simulink model "CONTROL_SYSTEM_V2"  (R2024a)
settings: Solver=ode1  StartTime=0.0  StopTime=inf  FixedStep=0.01  RelTol=1e-5
values from neighbouring files (symbols this model uses):
  B_aet = 0.1503    [System_Setting.m]
  Beta1 = 3*Omega_o    (= 750)    [Control_Setting.m]
  Beta2 = 3*(Omega_o^2)    (= 187500)    [Control_Setting.m]
  Beta3 = (Omega_o^3)    (= 15625000)    [Control_Setting.m]
  F_so = 0.089    [System_Setting.m]
  J_aet = 0.0035    [System_Setting.m]
  K_sp = 0.0914    [System_Setting.m]
  omga_c = 100    [Control_Setting.m]
  roa = 0.24    [System_Setting.m]
  theta_o = 12    [System_Setting.m]
  Toa_ho = 0.3193    [System_Setting.m]
undefined symbols (not defined in the file or in its folder): Desire_Max, Desire_Min, Direction_Pin, EN_Pin, Kd, Ki, Kn, Kp, sigbuilder_block
libraries: arduinolib x29, simulink_extras x12, slpidlib x3, spsOnDelayLib x2, simulink x2, slctrl_autotuning x2
(part 1 of 3)
settings Model: NumberOfSteps=2  ExtModeTrigDuration=2  Creator=Banana444  LastModifiedBy=Banana444
settings SolverCC: ZeroCrossAlgorithm=Adaptive  AutoInsertRateTranBlk=on
settings OptimizationCC: EnhancedBackFolding=on  PassReuseOutputArgsAs=Individual arguments  ZeroExternalMemoryAtStartup=off  ZeroInternalMemoryAtStartup=off  MaxStackSize=64  OptimizeBlockOrder=speed  DifferentSizesBufferReuse=on  OptimizationCustomize=off  EfficientTunableParamExpr=on
settings DebuggingCC: IgnoredZcDiagnostic=none  ParameterTunabilityLossMsg=error
settings HardwareCC: ProdBitPerPointer=32  ProdBitPerSizeT=32  ProdBitPerPtrDiffT=32  ProdLargestAtomicInteger=Long  ProdLargestAtomicFloat=Double  ProdWordSize=32  ProdHWDeviceType=ARM Compatible->ARM Cortex
settings SFSimCC: MATLABDynamicMemAlloc=off
settings RTWCC: Description=Embedded Coder  SystemTargetFile=ert.tlc  HardwareBoard=ESP32-WROOM(Arduino Compatible)  TLCOptions="-aInlineSetEventsForThisBaseRateFcn=TLC_FALSE -aSuppressMultiTaskScheduler=TLC_FALSE  -aRateBasedStepFcn=0"  TemplateMakefile=ert_default_tmf  Toolchain=ESP32
settings CodeAppCC: ForceParamTrailComments=on  IgnoreCustomStorageClasses=off  OperatorAnnotations=on  SimulinkDataObjDesc=on  SFDataObjDesc=on  InsertBlockDesc=on
settings ERTTargetCC: SupportContinuousTime=on  SupportVariableSizeSignals=on  ExtModeTransport=3  ExtModeStaticAlloc=on  ExtModeAutomaticAllocSize=off  ExtModeStaticAllocSize=65536  ExtModeMexFile=ext_xcp  ExtModeIntrfLevel=Level2 - Open

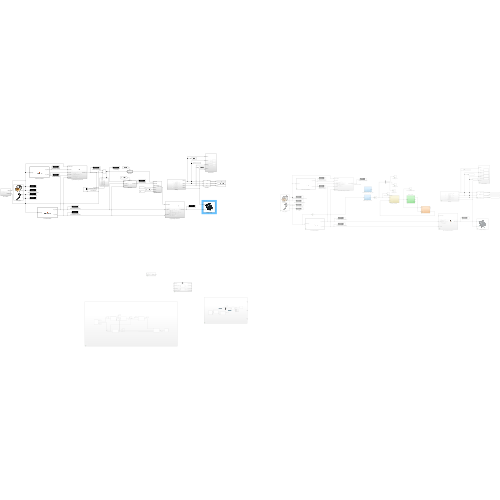
[thumbnail: Simulink's stored preview of the top-level diagram]
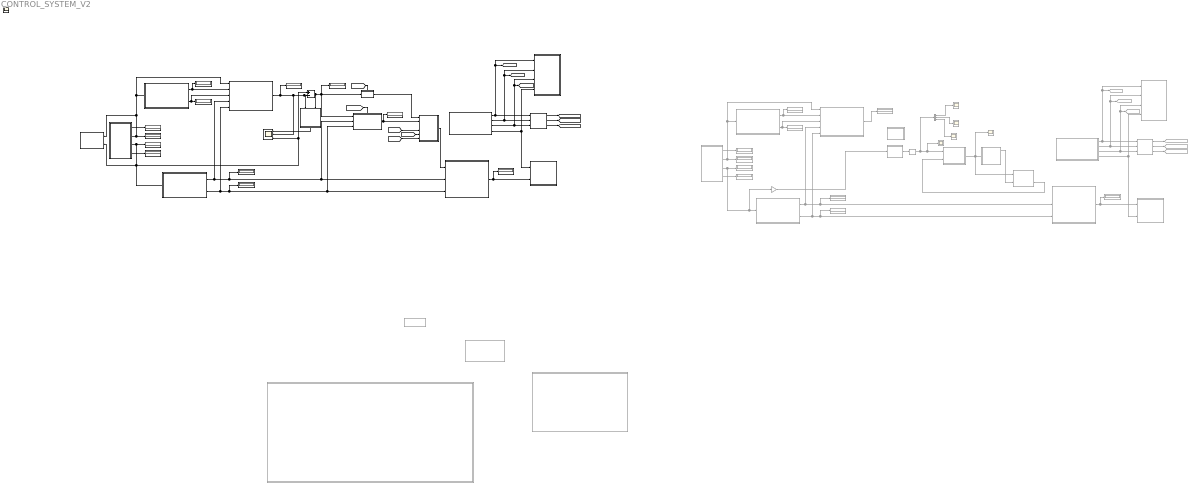
== system CONTROL_SYSTEM_V2 ==
  AETV_system : Subsystem  Commented=on
  Analog Signal : Subsystem
      mask Display: image('Capture.JPG');
  Analog Signal1 : Subsystem  Commented=on
      mask Display: image('Capture.JPG');
  Button Control : Subsystem
  Button Control1 : Subsystem  Commented=on
  Contro_input (Voltages) : Scope  Commented=on
  Contro_input (Voltages)1 : Scope  Commented=on
  Degrees to Radians1 : simulink_extras/Transformations/Degrees to Radians  Commented=on
  Demux : Demux  Commented=on  Outputs=3
  Desired signals_Sinewave : Subsystem  Commented=on
  Desired_Reference_step_input : Subsystem  Commented=on
  Display1 : Display  Commented=on
      settings: Decimation=2
  Display3 : Display
      settings: Decimation=2
  Error Indication : Subsystem
      settings: PortSchema="{\"entries\":[{\"content\":{\"sides\":[{\"content\":{},\"type\":\"ConnectorPlacement.EquallySpacedRectSide\",\"uuid\":\"6bb27259-0fc4-412b-bd28-187413250838\"},{\"content\":{\"connectorIds\":[\"In1\",\"In2\"],\"side\":\"RIGHT\"},\"type\":\"ConnectorPlacement.EquallySpacedRectSide\",\"uuid\":\"b38a583a-7cdb-4b72-8a0e-445370b0f03f\"},{\"content\":{\"side\":\"TOP\"},\"type\":\"ConnectorPlacement.EquallySpacedRectSide\",\"uuid\":\"477ad40e-8e68-4653-afaf-50b4ab734c9d\"}]},\"type\":\"ConnectorPlacement.EquallySpacedConnector\",\"uuid\":\"474c0f68-6b48-44ee-b6ec-af4e49acdc40\"}],\"packageUris\":[\"http://schema.mathworks.com/mf0/Connector/R2020b\"],\"version\":\"1.0\"}"
  Error Reading : Display
      settings: Decimation=2
  FP_Input Range Conversion : Subsystem
  FP_Input Range Conversion1 : Subsystem  Commented=on
  Foot Pedal Calibration : MATLAB Function  TreatAsAtomicUnit=on
  Foot Pedal Calibration1 : MATLAB Function  Commented=on  TreatAsAtomicUnit=on
  Foot Pedal Maximum Reading : Display
      settings: Decimation=2
  Foot Pedal Maximum Reading1 : Display  Commented=on
      settings: Decimation=2
  Foot Pedal Minimum Reading : Display
      settings: Decimation=2
  Foot Pedal Minimum Reading1 : Display  Commented=on
      settings: Decimation=2
  Foot Pedal Reading : Display
      settings: Decimation=2
  Foot Pedal Reading1 : Display  Commented=on
      settings: Decimation=2
  Foot Pedal Signal VS Throttle Body Position : Scope  NumInputPorts=3
  Goto10 : Goto  Commented=on  GotoTag=Button_2
  Goto11 : Goto  Commented=on  GotoTag=Button_3
  Goto6 : Goto  Commented=on  GotoTag=No_Control
  Goto7 : Goto  Commented=on  GotoTag=PID_Control
  Goto8 : Goto  Commented=on  GotoTag=Advance_Control
  Goto9 : Goto  Commented=on  GotoTag=Button_1
  H-Bridge Setting : Subsystem
      mask Display: image('H-Bridge-removebg-preview.png');
  H-Bridge Setting1 : Subsystem  Commented=on
      mask Display: image('H-Bridge-removebg-preview.png');
  If Condition : If  NumInputs=3  IfExpression=u1 == 1  ElseIfExpressions=u2 == 1, u3 == 1  ShowElse=off
  If Condition1 : If  Commented=on  NumInputs=3  IfExpression=u1 == 1  ElseIfExpressions=u2 == 1, u3 == 1  ShowElse=off
  Latching : Subsystem
  Latching1 : Subsystem  Commented=on
  Multiply : Gain  Commented=on  Gain=10
  NaN : Display
      settings: Decimation=2
  NaN1 : Display  Commented=on
      settings: Decimation=2
  No Control : Subsystem  TreatAsAtomicUnit=on
  Operation Selector : Subsystem
  PID Control : Subsystem
  PID Output Reading : Display
      settings: Decimation=2
  SFBC_Controller : Subsystem  Commented=on
  Subsystem : Subsystem
      settings: PortSchema="{\"entries\":[{\"content\":{\"sides\":[{\"content\":{},\"type\":\"ConnectorPlacement.EquallySpacedRectSide\",\"uuid\":\"06ab9b8c-dc11-4e78-9aea-2a49b899d383\"},{\"content\":{\"side\":\"RIGHT\"},\"type\":\"ConnectorPlacement.EquallySpacedRectSide\",\"uuid\":\"ea81575a-6f3e-44ea-98d6-a15110b05ea2\"},{\"content\":{\"connectorIds\":[\"In1\",\"In2\"],\"side\":\"TOP\"},\"type\":\"ConnectorPlacement.EquallySpacedRectSide\",\"uuid\":\"b4582e74-93d2-4cba-bd7b-a3215d2fef1c\"},{\"content\":{\"connectorIds\":[\"Out1\"],\"side\":\"BOTTOM\"},\"type\":\"ConnectorPlacement.EquallySpacedRectSide\",\"uuid\":\"d3012ec7-4a68-4cee-bd0d-e63c4f089545\"}]},\"type\":\"ConnectorPlacement.EquallySpacedConnector\",\"uuid\":\"85ff3d74-6a46-44e9-8a38-f9999c5d3ee8\"}],\"packageUris\":[\"http://schema.mathworks.com/mf0/Connector/R2020b\"],\"version\":\"1.0\"}"
  Subsystem1 : Subsystem  Commented=on
  Subsystem2 : Subsystem  Commented=on
  Subsystem4 : Subsystem  Commented=on
  Subsystem5 : Subsystem  Commented=on
  Subsystem6 : Subsystem  Commented=on
  Sum2 : Sum  Inputs=+-
  TB Maximum Reading : Display
      settings: Decimation=2
  TB Maximum Reading1 : Display  Commented=on
      settings: Decimation=2
  TB Minimum Reading : Display
      settings: Decimation=2
  TB Minimum Reading1 : Display  Commented=on
      settings: Decimation=2
  TB New Range Reading : Display
      settings: Decimation=2
  TB New Range Reading1 : Display  Commented=on
      settings: Decimation=2
  TB_Feedbakc Range Conversion : Subsystem
  TB_Feedbakc Range Conversion1 : Subsystem  Commented=on
  Throttle Body Callibration : MATLAB Function  TreatAsAtomicUnit=on
  Throttle Body Callibration1 : MATLAB Function  Commented=on  TreatAsAtomicUnit=on
  Throttle Body Feeback Reading : Display
      settings: Decimation=2
  Throttle Body Feeback Reading (Unused) : Display
      settings: Decimation=2
  Throttle Body Feeback Reading (Unused)1 : Display  Commented=on
      settings: Decimation=2
  Throttle Body Feeback Reading1 : Display  Commented=on
      settings: Decimation=2
  Tracking erro1 : Scope  Commented=on
  Tracking erro2 : Scope  Commented=on
  Tracking erro3 : Scope  Commented=on
  Scope1 : Scope
  wires:
  Analog Signal/4(Out4) -> NaN/1
  Foot Pedal Calibration/1(FP_maxVal) -> FP_Input Range Conversion/2(FP_maxVal), PID Control/2(FP_maxVal), Foot Pedal Maximum Reading/1, TB_Feedbakc Range Conversion/4(FP_maxVal)
  [PID_Control] -> PID Control/Action
  Analog Signal/1(Out1) -> Throttle Body Feeback Reading (Unused)/1
  Analog Signal/2(TBRange) -> Throttle Body Feeback Reading/1, Error Indication/1(TBRange), Throttle Body Callibration/1(TB_Range), TB_Feedbakc Range Conversion/1(Control Output)
  Analog Signal/3(PedalRange) -> Foot Pedal Reading/1, Sum2/1, Foot Pedal Signal VS Throttle Body Position/3, Error Indication/2(PedalRange), Foot Pedal Calibration/1(PedalRange)  "Foot Pedal Signal"
  Foot Pedal Calibration/2(FP_minVal) -> FP_Input Range Conversion/3(FP_minVal), PID Control/3(FP_minVal), Foot Pedal Minimum Reading/1, TB_Feedbakc Range Conversion/5(FP_minVal)
  [No_Control] -> No Control/Action
  Operation Selector/1(Control Output) -> FP_Input Range Conversion/1(Control Output)
  If Condition/2 -> [PID_Control]
  TB_Feedbakc Range Conversion/1(TB New Range) -> Sum2/2, Subsystem/1(Throttle Body Feedback), Foot Pedal Signal VS Throttle Body Position/2, TB New Range Reading/1  "Throttle Body Feedback"
  PID Control/1(PID Output) -> Operation Selector/2(PID Output), PID Output Reading/1
  FP_Input Range Conversion/1(0 - 255 Output) -> H-Bridge Setting/2(0 - 255), Display3/1
  Sum2/1 -> No Control/1(In1), PID Control/1(Error), Error Reading/1, Subsystem/2(In1)  "Error"
  If Condition/1 -> [No_Control]
  Throttle Body Callibration/1(TB_maxVal) -> TB Maximum Reading/1, TB_Feedbakc Range Conversion/2(TB_maxVal)
  Throttle Body Callibration/2(TB_minVal) -> TB Minimum Reading/1, TB_Feedbakc Range Conversion/3(TB_minVal)
  Latching/4(Button 4) -> H-Bridge Setting/1(Calibration Mode), Button Control/4(Button 4)
  Latching/3(Button 3) -> If Condition/3, [Button_3], Button Control/3(Button 3)
  Latching/1(Button 1) -> [Button_1], Button Control/1(Button 1), If Condition/1
  If Condition/3 -> [Advance_Control]
  Latching/2(Button 2) -> [Button_2], Button Control/2(Bottun 2), If Condition/2
  [Button_1] -> Operation Selector/4(Switch 1)
  [Button_2] -> Operation Selector/5(Switch 2)
  [Button_3] -> Operation Selector/6(Switch 3)
  No Control/1(Out1) -> Operation Selector/1(No Control)
  Latching1/2(Out2) -> Goto10/1, Button Control1/2(Bottun 2), If Condition1/2
  If Condition1/3 -> Goto8/1
  Latching1/4(Out4) -> H-Bridge Setting1/2(Calibration Mode), Button Control1/4(Button 4)
  Analog Signal1/4(Out4) -> NaN1/1
  Throttle Body Callibration1/2(TB_minVal) -> TB Minimum Reading1/1, TB_Feedbakc Range Conversion1/3(TB_minVal)
  Latching1/3(Out3) -> If Condition1/3, Goto11/1, Button Control1/3(Button 3)
  FP_Input Range Conversion1/1(0 - 255 Output) -> H-Bridge Setting1/1(0 - 255), Display1/1
  TB_Feedbakc Range Conversion1/1(TB New Range) -> TB New Range Reading1/1  "Throttle Body Feedback"
  Foot Pedal Calibration1/1(FP_maxVal) -> FP_Input Range Conversion1/2(FP_maxVal), Foot Pedal Maximum Reading1/1, TB_Feedbakc Range Conversion1/4(FP_maxVal)
  Foot Pedal Calibration1/2(FP_minVal) -> FP_Input Range Conversion1/3(FP_minVal), Foot Pedal Minimum Reading1/1, TB_Feedbakc Range Conversion1/5(FP_minVal)
  Throttle Body Callibration1/1(TB_maxVal) -> TB Maximum Reading1/1, TB_Feedbakc Range Conversion1/2(TB_maxVal)
  Analog Signal1/1(Out1) -> Throttle Body Feeback Reading (Unused)1/1
  If Condition1/2 -> Goto7/1
  Analog Signal1/3(PedalRange) -> Foot Pedal Reading1/1, Multiply/1, Foot Pedal Calibration1/1(PedalRange)  "Foot Pedal Signal"
  Latching1/1(Out1) -> Goto9/1, Button Control1/1(Button 1), If Condition1/1
  Analog Signal1/2(TBRange) -> Throttle Body Feeback Reading1/1, Throttle Body Callibration1/1(TB_Range), TB_Feedbakc Range Conversion1/1(Control Output)
  If Condition1/1 -> Goto6/1
  Subsystem5/2(Xi^) -> SFBC_Controller/2(Xi^)
  Desired signals_Sinewave/1(xi_d) -> Degrees to Radians1/1
  SFBC_Controller/1(Out1) -> Subsystem5/1(U(t)), AETV_system/1(U(t)), Contro_input (Voltages)/1
  AETV_system/1(X1) -> Subsystem5/2(X1(t))
  Multiply/1 -> Desired signals_Sinewave/1(Input)
  Demux/2 -> Tracking erro2/1
  Degrees to Radians1/1 -> Demux/1, SFBC_Controller/1(Xd_i), Contro_input (Voltages)1/1
  Demux/3 -> Tracking erro3/1
  Demux/1 -> Tracking erro1/1
  Subsystem/1(Percentage Error) -> Foot Pedal Signal VS Throttle Body Position/1  "Percentage Error"

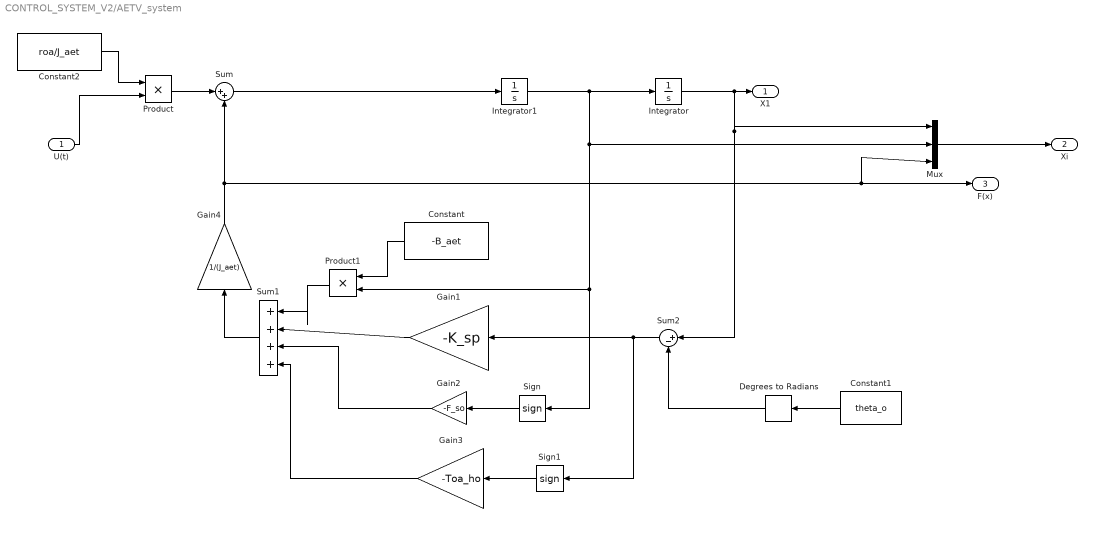
== system CONTROL_SYSTEM_V2/AETV_system ==
  U(t) : Inport
  Constant : Constant  Value=-B_aet
  Constant1 : Constant  Value=theta_o
  Constant2 : Constant  Value=roa/J_aet
  Degrees to Radians : simulink_extras/Transformations/Degrees to Radians
  Gain1 : Gain  Gain=-K_sp
  Gain2 : Gain  Gain=-F_so
  Gain3 : Gain  Gain=-Toa_ho
  Gain4 : Gain  Gain=1/(J_aet)
  Integrator : Integrator  InitialCondition=12*pi/180
  Integrator1 : Integrator
  Mux : Mux  Inputs=3
  Product : Product  RndMeth=Zero
  Product1 : Product  RndMeth=Zero
  Sign : Signum
  Sign1 : Signum
  Sum : Sum  Inputs=|++
  Sum1 : Sum  Inputs=|++++
  Sum2 : Sum  Inputs=|+-
  X1 : Outport
  Xi : Outport  Port=2
  F(x) : Outport  Port=3
  wires:
  Integrator1/1 -> Integrator/1, Product1/2, Sign/1, Mux/2
  Integrator/1 -> Sum2/1, Mux/1, X1/1
  Sum1/1 -> Gain4/1
  Constant/1 -> Product1/1
  Product1/1 -> Sum1/1
  Gain1/1 -> Sum1/2
  Sign/1 -> Gain2/1
  Gain2/1 -> Sum1/3
  Constant1/1 -> Degrees to Radians/1
  Sum2/1 -> Sign1/1, Gain1/1
  Gain3/1 -> Sum1/4
  Sign1/1 -> Gain3/1
  Sum/1 -> Integrator1/1
  Product/1 -> Sum/1
  Constant2/1 -> Product/1
  U(t)/1 -> Product/2
  Mux/1 -> Xi/1
  Gain4/1 -> Sum/2, Mux/3, F(x)/1
  Degrees to Radians/1 -> Sum2/2

== system CONTROL_SYSTEM_V2/Analog Signal ==
  note: Analog Read Custom Block reaading;
      | - Throttle Body Feedback (V1)
      | - Foot Padel Signal (V2)
  MATLAB System : MATLABSystem  System=ADS1115_Vread  SetGain=int16( 16 )  SampleTime=-1
      mask Type: ADS1115_Vread
      mask Display:
      | color('white');plot([100,100,100,100]*1,[100,100,100,100]*1);plot([100,100,100,100]*0,[100,100,100,100]*0);color('blue');text(38, 92, 'IO Device Builder','horizontalAlignment', 'right');
      | color('black');text(52,50,' ADS1115_Vread','horizontalAlignment','center');
      | port_label('output',1,'V0');port_label('output',2,'V1');port_label('output',3,'V2');port_label('output',4,'V3');
  Out1 : Outport
  TBRange : Outport  Port=2
  PedalRange : Outport  Port=3
  Out4 : Outport  Port=4
  wires:
  MATLAB System/1 -> Out1/1
  MATLAB System/3 -> PedalRange/1
  MATLAB System/2 -> TBRange/1
  MATLAB System/4 -> Out4/1

== system CONTROL_SYSTEM_V2/Analog Signal1 ==
  note: Analog Read Custom Block reaading;
      | - Throttle Body Feedback (V1)
      | - Foot Padel Signal (V2)
  MATLAB System : MATLABSystem  System=ADS1115_Vread  SetGain=int16( 16 )  SampleTime=-1
      mask Type: ADS1115_Vread
      mask Display:
      | color('white');plot([100,100,100,100]*1,[100,100,100,100]*1);plot([100,100,100,100]*0,[100,100,100,100]*0);color('blue');text(38, 92, 'IO Device Builder','horizontalAlignment', 'right');
      | color('black');text(52,50,' ADS1115_Vread','horizontalAlignment','center');
      | port_label('output',1,'V0');port_label('output',2,'V1');port_label('output',3,'V2');port_label('output',4,'V3');
  Out1 : Outport
  TBRange : Outport  Port=2
  PedalRange : Outport  Port=3
  Out4 : Outport  Port=4
  wires:
  MATLAB System/1 -> Out1/1
  MATLAB System/3 -> PedalRange/1
  MATLAB System/2 -> TBRange/1
  MATLAB System/4 -> Out4/1

== system CONTROL_SYSTEM_V2/Button Control ==
  Button 1 : Inport
  Bottun 2 : Inport  Port=2
  Button 3 : Inport  Port=3
  Button 4 : Inport  Port=4
  Constant : Constant  Value=0
  Digital Output : arduinolib/Digital Output  pinNumber=27  Direction=output  blockPlatform=arduino
  Digital Output1 : arduinolib/Digital Output  pinNumber=26  Direction=output  blockPlatform=arduino
  Digital Output2 : arduinolib/Digital Output  pinNumber=25  Direction=output  blockPlatform=arduino
  Digital Output3 : arduinolib/Digital Output  pinNumber=33  Direction=output  blockPlatform=arduino
  Pulse Generator : DiscretePulseGenerator  PulseType=Time based  Period=0.5  PulseWidth=50
  Switch : Switch  Criteria=u2 ~= 0  SaturateOnIntegerOverflow=off  InputSameDT=off
  wires:
  Button 1/1 -> Digital Output/1
  Bottun 2/1 -> Digital Output1/1
  Button 3/1 -> Digital Output2/1
  Pulse Generator/1 -> Switch/1
  Button 4/1 -> Switch/2
  Constant/1 -> Switch/3
  Switch/1 -> Digital Output3/1

== system CONTROL_SYSTEM_V2/Button Control1 ==
  Button 1 : Inport
  Bottun 2 : Inport  Port=2
  Button 3 : Inport  Port=3
  Button 4 : Inport  Port=4
  Digital Output : arduinolib/Digital Output  pinNumber=27  Direction=output  blockPlatform=arduino
  Digital Output1 : arduinolib/Digital Output  pinNumber=26  Direction=output  blockPlatform=arduino
  Digital Output2 : arduinolib/Digital Output  pinNumber=25  Direction=output  blockPlatform=arduino
  Digital Output3 : arduinolib/Digital Output  pinNumber=33  Direction=output  blockPlatform=arduino
  wires:
  Button 1/1 -> Digital Output/1
  Bottun 2/1 -> Digital Output1/1
  Button 3/1 -> Digital Output2/1
  Button 4/1 -> Digital Output3/1

== system CONTROL_SYSTEM_V2/Desired signals_Sinewave ==
  Input : Inport
  Fcn1 : Fcn  Expr=10*sin(2*u)+10+7
  Fcn2 : Fcn  Expr=10*2*cos(2*u)
  Fcn3 : Fcn  Expr=-10*2*2*sin(2*u)
  Input1 : InportShadow
  Input2 : InportShadow
  Mux : Mux  Inputs=3
  xi_d : Outport
  wires:
  Input/1 -> Fcn1/1
  Input1/1 -> Fcn2/1
  Input2/1 -> Fcn3/1
  Fcn1/1 -> Mux/1
  Fcn2/1 -> Mux/2
  Fcn3/1 -> Mux/3
  Mux/1 -> xi_d/1

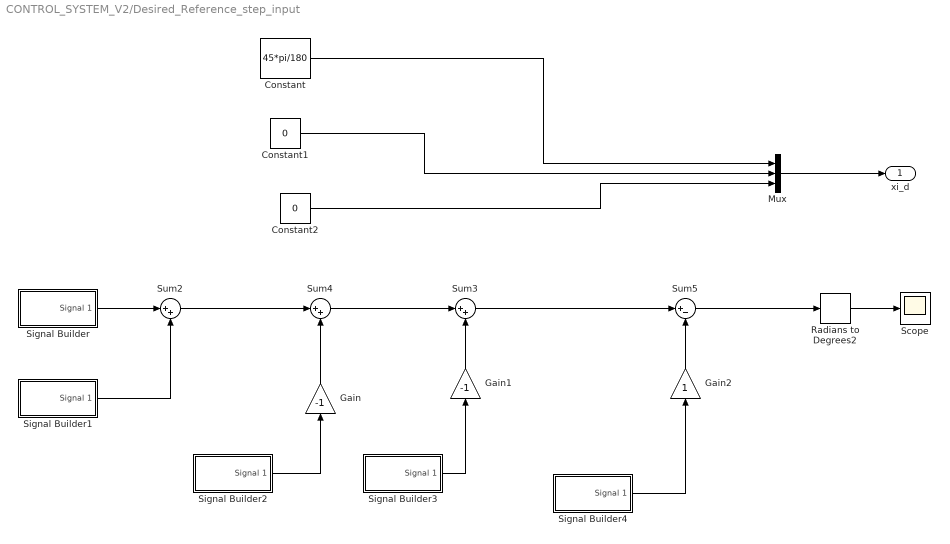
== system CONTROL_SYSTEM_V2/Desired_Reference_step_input ==
  Constant : Constant  Value=45*pi/180
  Constant1 : Constant  Value=0
  Constant2 : Constant  Value=0
  Gain : Gain  Gain=-1
  Gain1 : Gain  Gain=-1
  Gain2 : Gain
  Mux : Mux  Inputs=3
  Radians to Degrees2 : simulink_extras/Transformations/Radians to Degrees
  Scope : Scope
  Signal Builder : Subsystem  Tag=STV Subsys  LoadFcn=sigbuilder_block('load');  StartFcn=sigbuilder_block('start');  StopFcn=sigbuilder_block('stop');  ClipboardFcn=sigbuilder_block('clipboard');  mask(Sigbuilder block){tuvar=[0:10]}
      mask help: Create and generate interchangeable groups of signals whose waveforms are piecewise linear.
      mask init:
      | if ~strcmp(get_param(bdroot(gcbh),'SimulationStatus'),'stopped') tuvar = sigbuilder_block('maskInit'); end
      settings: CopyFcn=sigbuilder_block('copy');  DeleteFcn=sigbuilder_block('delete');  ModelCloseFcn=sigbuilder_block('modelClose');  PreSaveFcn=sigbuilder_block('preSave');  PauseFcn=sigbuilder_block('pause')  ContinueFcn=sigbuilder_block('continue')  NameChangeFcn=sigbuilder_block('namechange');  OpenFcn=sigbuilder_block('open',[437.25 117.75 550.5 394.5 ]);  CloseFcn=sigbuilder_block('close');
      mask Display: plot(0, 0, 100, 100,[2, 2, 32, 32, 2], [68, 8, 8, 68, 68],[32, 2], [38, 38], [32, 19, 2],[53, 60, 44], [32, 17, 17, 2],[16, 16, 31, 31]);txt = getActiveGroup(gcbh);text(2, 100, txt,'verticalAlignment', 'top');
  Signal Builder1 : Subsystem  Tag=STV Subsys  LoadFcn=sigbuilder_block('load');  StartFcn=sigbuilder_block('start');  StopFcn=sigbuilder_block('stop');  ClipboardFcn=sigbuilder_block('clipboard');  mask(Sigbuilder block){tuvar=[0:10]}
      mask help: Create and generate interchangeable groups of signals whose waveforms are piecewise linear.
      mask init:
      | if ~strcmp(get_param(bdroot(gcbh),'SimulationStatus'),'stopped') tuvar = sigbuilder_block('maskInit'); end
      settings: CopyFcn=sigbuilder_block('copy');  DeleteFcn=sigbuilder_block('delete');  ModelCloseFcn=sigbuilder_block('modelClose');  PreSaveFcn=sigbuilder_block('preSave');  PauseFcn=sigbuilder_block('pause')  ContinueFcn=sigbuilder_block('continue')  NameChangeFcn=sigbuilder_block('namechange');  OpenFcn=sigbuilder_block('open',[437.25 117.75 550.5 394.5 ]);  CloseFcn=sigbuilder_block('close');
      mask Display: plot(0, 0, 100, 100,[2, 2, 32, 32, 2], [68, 8, 8, 68, 68],[32, 2], [38, 38], [32, 19, 2],[53, 60, 44], [32, 17, 17, 2],[16, 16, 31, 31]);txt = getActiveGroup(gcbh);text(2, 100, txt,'verticalAlignment', 'top');
  Signal Builder2 : Subsystem  Tag=STV Subsys  LoadFcn=sigbuilder_block('load');  StartFcn=sigbuilder_block('start');  StopFcn=sigbuilder_block('stop');  ClipboardFcn=sigbuilder_block('clipboard');  mask(Sigbuilder block){tuvar=[0:10]}
      mask help: Create and generate interchangeable groups of signals whose waveforms are piecewise linear.
      mask init:
      | if ~strcmp(get_param(bdroot(gcbh),'SimulationStatus'),'stopped') tuvar = sigbuilder_block('maskInit'); end
      settings: CopyFcn=sigbuilder_block('copy');  DeleteFcn=sigbuilder_block('delete');  ModelCloseFcn=sigbuilder_block('modelClose');  PreSaveFcn=sigbuilder_block('preSave');  PauseFcn=sigbuilder_block('pause')  ContinueFcn=sigbuilder_block('continue')  NameChangeFcn=sigbuilder_block('namechange');  OpenFcn=sigbuilder_block('open',[437.25 117.75 550.5 394.5 ]);  CloseFcn=sigbuilder_block('close');
      mask Display: plot(0, 0, 100, 100,[2, 2, 32, 32, 2], [68, 8, 8, 68, 68],[32, 2], [38, 38], [32, 19, 2],[53, 60, 44], [32, 17, 17, 2],[16, 16, 31, 31]);txt = getActiveGroup(gcbh);text(2, 100, txt,'verticalAlignment', 'top');
  Signal Builder3 : Subsystem  Tag=STV Subsys  LoadFcn=sigbuilder_block('load');  StartFcn=sigbuilder_block('start');  StopFcn=sigbuilder_block('stop');  ClipboardFcn=sigbuilder_block('clipboard');  mask(Sigbuilder block){tuvar=[0:10]}
      mask help: Create and generate interchangeable groups of signals whose waveforms are piecewise linear.
      mask init:
      | if ~strcmp(get_param(bdroot(gcbh),'SimulationStatus'),'stopped') tuvar = sigbuilder_block('maskInit'); end
      settings: CopyFcn=sigbuilder_block('copy');  DeleteFcn=sigbuilder_block('delete');  ModelCloseFcn=sigbuilder_block('modelClose');  PreSaveFcn=sigbuilder_block('preSave');  PauseFcn=sigbuilder_block('pause')  ContinueFcn=sigbuilder_block('continue')  NameChangeFcn=sigbuilder_block('namechange');  OpenFcn=sigbuilder_block('open',[437.25 117.75 550.5 394.5 ]);  CloseFcn=sigbuilder_block('close');
      mask Display: plot(0, 0, 100, 100,[2, 2, 32, 32, 2], [68, 8, 8, 68, 68],[32, 2], [38, 38], [32, 19, 2],[53, 60, 44], [32, 17, 17, 2],[16, 16, 31, 31]);txt = getActiveGroup(gcbh);text(2, 100, txt,'verticalAlignment', 'top');
  Signal Builder4 : Subsystem  Tag=STV Subsys  LoadFcn=sigbuilder_block('load');  StartFcn=sigbuilder_block('start');  StopFcn=sigbuilder_block('stop');  ClipboardFcn=sigbuilder_block('clipboard');  mask(Sigbuilder block){tuvar=[0:10]}
      mask help: Create and generate interchangeable groups of signals whose waveforms are piecewise linear.
      mask init:
      | if ~strcmp(get_param(bdroot(gcbh),'SimulationStatus'),'stopped') tuvar = sigbuilder_block('maskInit'); end
      settings: CopyFcn=sigbuilder_block('copy');  DeleteFcn=sigbuilder_block('delete');  ModelCloseFcn=sigbuilder_block('modelClose');  PreSaveFcn=sigbuilder_block('preSave');  PauseFcn=sigbuilder_block('pause')  ContinueFcn=sigbuilder_block('continue')  NameChangeFcn=sigbuilder_block('namechange');  OpenFcn=sigbuilder_block('open',[437.25 117.75 550.5 394.5 ]);  CloseFcn=sigbuilder_block('close');
      mask Display: plot(0, 0, 100, 100,[2, 2, 32, 32, 2], [68, 8, 8, 68, 68],[32, 2], [38, 38], [32, 19, 2],[53, 60, 44], [32, 17, 17, 2],[16, 16, 31, 31]);txt = getActiveGroup(gcbh);text(2, 100, txt,'verticalAlignment', 'top');
  Sum2 : Sum  Inputs=|++
  Sum3 : Sum  Inputs=|++
  Sum4 : Sum  Inputs=|++
  Sum5 : Sum  Inputs=|+-
  xi_d : Outport
  wires:
  Signal Builder/1(Signal 1) -> Sum2/1
  Signal Builder1/1(Signal 1) -> Sum2/2
  Sum2/1 -> Sum4/1
  Signal Builder2/1(Signal 1) -> Gain/1
  Gain/1 -> Sum4/2
  Sum4/1 -> Sum3/1
  Signal Builder3/1(Signal 1) -> Gain1/1
  Gain1/1 -> Sum3/2
  Sum3/1 -> Sum5/1
  Signal Builder4/1(Signal 1) -> Gain2/1
  Gain2/1 -> Sum5/2
  Sum5/1 -> Radians to Degrees2/1
  Radians to Degrees2/1 -> Scope/1
  Constant/1 -> Mux/1
  Mux/1 -> xi_d/1
  Constant1/1 -> Mux/2
  Constant2/1 -> Mux/3

== system CONTROL_SYSTEM_V2/Error Indication ==
  TBRange : Inport
  PedalRange : Inport  Port=2
  Constant : Constant
  Constant1 : Constant  Value=0
  Constant2 : Constant
  Constant3 : Constant  Value=0
  Constant4 : Constant  Value=0
  Digital Output4 : arduinolib/Digital Output  pinNumber=32  Direction=output  blockPlatform=arduino
  OR : Logic  Operator=NAND  IconShape=distinctive  AllPortsSameDT=off  OutDataTypeStr=boolean
  Pulse Generator : DiscretePulseGenerator  PulseType=Time based  Period=0.1  PulseWidth=50
  Switch : Switch  Criteria=u2 > Threshold  SaturateOnIntegerOverflow=off  InputSameDT=off
  Switch2 : Switch  Criteria=u2 > Threshold  SaturateOnIntegerOverflow=off  InputSameDT=off
  Switch3 : Switch  Criteria=u2 > Threshold  SaturateOnIntegerOverflow=off  InputSameDT=off
  wires:
  Switch3/1 -> Digital Output4/1
  Pulse Generator/1 -> Switch3/1
  Constant3/1 -> Switch2/3
  Switch/1 -> OR/1
  Switch2/1 -> OR/2
  Constant2/1 -> Switch2/1
  Constant/1 -> Switch/1
  Constant1/1 -> Switch/3
  OR/1 -> Switch3/2
  PedalRange/1 -> Switch2/2
  TBRange/1 -> Switch/2
  Constant4/1 -> Switch3/3

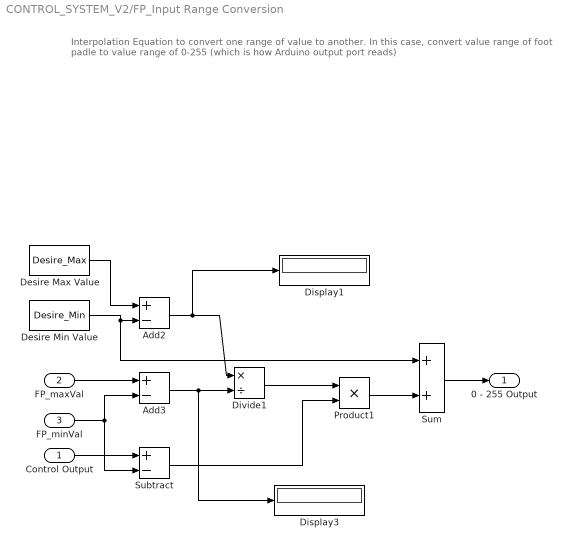
== system CONTROL_SYSTEM_V2/FP_Input Range Conversion ==
  note: Interpolation Equation to convert one range of value to another.
      | In this case, convert value range of foot padle to value range of 0-255 (which is how Arduino output port reads)
  Control Output : Inport
  FP_maxVal : Inport  Port=2
  FP_minVal : Inport  Port=3
  Add2 : Sum  Inputs=+-
  Add3 : Sum  Inputs=+-
  Desire Max Value : Constant  Value=Desire_Max
  Desire Min Value : Constant  Value=Desire_Min
  Display1 : Display
  Display3 : Display
  Divide1 : Product  Inputs=*/
  Product1 : Product
  Subtract : Sum  Inputs=+-
  Sum : Sum
  0 - 255 Output : Outport
  wires:
  Control Output/1 -> Subtract/1
  FP_maxVal/1 -> Add3/1
  Add3/1 -> Divide1/2, Display3/1
  FP_minVal/1 -> Subtract/2, Add3/2
  Desire Min Value/1 -> Add2/2, Sum/1
  Subtract/1 -> Product1/2
  Desire Max Value/1 -> Add2/1
  Add2/1 -> Display1/1, Divide1/1
  Divide1/1 -> Product1/1
  Product1/1 -> Sum/2
  Sum/1 -> 0 - 255 Output/1

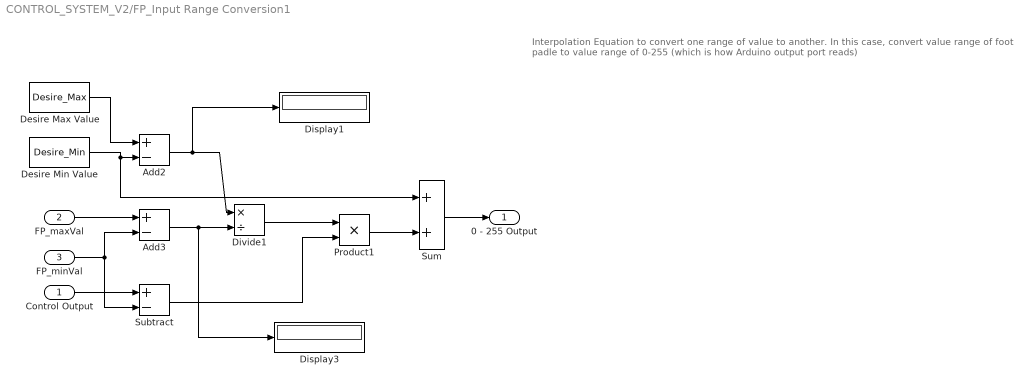
== system CONTROL_SYSTEM_V2/FP_Input Range Conversion1 ==
  note: Interpolation Equation to convert one range of value to another.
      | In this case, convert value range of foot padle to value range of 0-255 (which is how Arduino output port reads)
  Control Output : Inport
  FP_maxVal : Inport  Port=2
  FP_minVal : Inport  Port=3
  Add2 : Sum  Inputs=+-
  Add3 : Sum  Inputs=+-
  Desire Max Value : Constant  Value=Desire_Max
  Desire Min Value : Constant  Value=Desire_Min
  Display1 : Display
  Display3 : Display
  Divide1 : Product  Inputs=*/
  Product1 : Product
  Subtract : Sum  Inputs=+-
  Sum : Sum
  0 - 255 Output : Outport
  wires:
  Control Output/1 -> Subtract/1
  FP_maxVal/1 -> Add3/1
  Add3/1 -> Divide1/2, Display3/1
  FP_minVal/1 -> Subtract/2, Add3/2
  Desire Min Value/1 -> Add2/2, Sum/1
  Subtract/1 -> Product1/2
  Desire Max Value/1 -> Add2/1
  Add2/1 -> Display1/1, Divide1/1
  Divide1/1 -> Product1/1
  Product1/1 -> Sum/2
  Sum/1 -> 0 - 255 Output/1

== system CONTROL_SYSTEM_V2/H-Bridge Setting ==
  note: The setup is for calibration the throttle body after pressing the calibration button (Button_4). This will force the throttle body to open for 2 seconds before it close
  note: Setting for H-Bridge to control the throttle body
      | Enable Pin = 0
      | Direction Pin = 1
  Calibration Mode : Inport
  0 - 255 : Inport  Port=2
  Constant : Constant  Value=0
  Digital Output : arduinolib/Digital Output  pinNumber=0  Direction=output  blockPlatform=arduino
  Digital Output1 : arduinolib/Digital Output  pinNumber=16  Direction=output  blockPlatform=arduino
  Direction Pin : Constant  Value=Direction_Pin
  Display3 : Display
  Display4 : Display
  Enable Pin : Constant  Value=EN_Pin
  Gain : Gain  Gain=100
  On Delay : spsOnDelayLib/On Delay  DelayType=On delay  delay=1  ic=0  Ts=0
  PWM : arduinolib/PWM  pinNumber=4  frequencyType=Specify  desiredFrequency=19000  achievableFrequency=19000
  Switch1 : Switch  Criteria=u2 ~= 0  SaturateOnIntegerOverflow=off  InputSameDT=off
  Switch2 : Switch  Criteria=u2 ~= 0  SaturateOnIntegerOverflow=off  InputSameDT=off
  wires:
  Enable Pin/1 -> Display4/1, Digital Output/1
  Direction Pin/1 -> Display3/1, Digital Output1/1
  Gain/1 -> Switch1/1
  Calibration Mode/1 -> On Delay/1, Switch1/2, Gain/1
  0 - 255/1 -> Switch1/3
  Switch1/1 -> Switch2/3
  Switch2/1 -> PWM/1
  On Delay/1 -> Switch2/2
  Constant/1 -> Switch2/1

== system CONTROL_SYSTEM_V2/H-Bridge Setting1 ==
  note: Setting for H-Bridge to control the throttle body
      | Enable Pin = 0
      | Direction Pin = 1
  0 - 255 : Inport
  Calibration Mode : Inport  Port=2
  Constant : Constant  Value=0
  Digital Output : arduinolib/Digital Output  pinNumber=0  Direction=output  blockPlatform=arduino
  Digital Output1 : arduinolib/Digital Output  pinNumber=16  Direction=output  blockPlatform=arduino
  Direction Pin : Constant  Value=Direction_Pin
  Display3 : Display
  Display4 : Display
  Enable Pin : Constant  Value=EN_Pin
  Gain : Gain  Gain=100
  On Delay : spsOnDelayLib/On Delay  DelayType=On delay  delay=2  ic=0  Ts=0
  PWM : arduinolib/PWM  pinNumber=4  frequencyType=Specify  desiredFrequency=19000  achievableFrequency=19000
  Switch1 : Switch  Criteria=u2 ~= 0  SaturateOnIntegerOverflow=off  InputSameDT=off
  Switch2 : Switch  Criteria=u2 ~= 0  SaturateOnIntegerOverflow=off  InputSameDT=off
  wires:
  Enable Pin/1 -> Display4/1, Digital Output/1
  Direction Pin/1 -> Display3/1, Digital Output1/1
  Gain/1 -> Switch1/1
  Calibration Mode/1 -> On Delay/1, Switch1/2, Gain/1
  0 - 255/1 -> Switch1/3
  Switch1/1 -> Switch2/3
  Switch2/1 -> PWM/1
  On Delay/1 -> Switch2/2
  Constant/1 -> Switch2/1

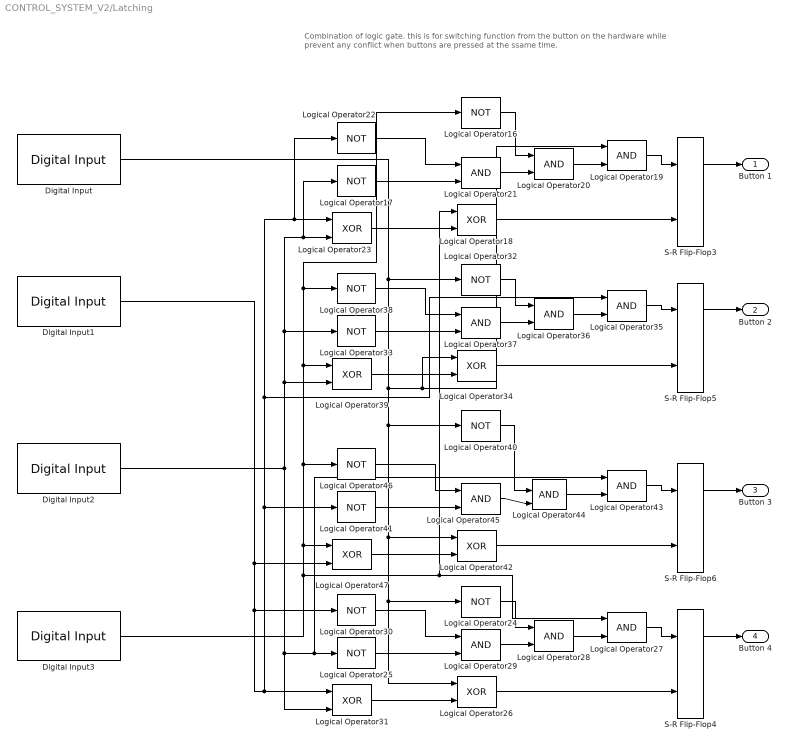
== system CONTROL_SYSTEM_V2/Latching ==
  note: Combination of logic gate. this is for switching function from the button on the hardware while prevent any conflict when buttons are pressed at the ssame time.
  Digital Input : arduinolib/Digital Input  pinNumber=36  mode=Default  Direction=input  SampleTime=-1  blockPlatform=arduino
  Digital Input1 : arduinolib/Digital Input  pinNumber=39  mode=Default  Direction=input  SampleTime=-1  blockPlatform=arduino
  Digital Input2 : arduinolib/Digital Input  pinNumber=34  mode=Default  Direction=input  SampleTime=-1  blockPlatform=arduino
  Digital Input3 : arduinolib/Digital Input  pinNumber=35  mode=Default  Direction=input  SampleTime=-1  blockPlatform=arduino
  Logical Operator{16..17,22,24..25,30,32..33,38,40..41,46} (12 alike) : Logic  Operator=NOT  IconShape=distinctive  AllPortsSameDT=off  OutDataTypeStr=boolean
  Logical Operator{18,23,26,31,34,39,42,47} (8 alike) : Logic  Operator=XOR  IconShape=distinctive  AllPortsSameDT=off  OutDataTypeStr=boolean
  Logical Operator{19..21,27..29,35..37,43..45} (12 alike) : Logic  IconShape=distinctive  AllPortsSameDT=off  OutDataTypeStr=boolean
  S-R Flip-Flop{3..6} (4 alike) : simulink_extras/Flip Flops/S-R Flip-Flop  initial_condition=0
  Button 1 : Outport
  Button 2 : Outport  Port=2
  Button 3 : Outport  Port=3
  Button 4 : Outport  Port=4
  wires:
  Digital Input2/1 -> Logical Operator25/1, Logical Operator43/1, Logical Operator31/2, Logical Operator17/1, Logical Operator23/2, Logical Operator33/1, Logical Operator39/2
  Digital Input3/1 -> Logical Operator16/1, Logical Operator38/1, Logical Operator39/1, Logical Operator46/1, Logical Operator47/1, Logical Operator18/1, Logical Operator27/1
  Digital Input1/1 -> Logical Operator47/2, Logical Operator30/1, Logical Operator41/1, Logical Operator22/1, Logical Operator23/1, Logical Operator35/1, Logical Operator31/1
  Logical Operator22/1 -> Logical Operator21/1
  Logical Operator17/1 -> Logical Operator21/2
  Logical Operator34/1 -> S-R Flip-Flop5/2
  Logical Operator33/1 -> Logical Operator37/2
  Logical Operator23/1 -> Logical Operator18/2
  Logical Operator39/1 -> Logical Operator34/2
  Logical Operator38/1 -> Logical Operator37/1
  Digital Input/1 -> Logical Operator40/1, Logical Operator24/1, Logical Operator26/1, Logical Operator42/1, Logical Operator19/1, Logical Operator34/1, Logical Operator32/1
  Logical Operator47/1 -> Logical Operator42/2
  Logical Operator46/1 -> Logical Operator45/1
  Logical Operator42/1 -> S-R Flip-Flop6/2
  Logical Operator41/1 -> Logical Operator45/2
  Logical Operator30/1 -> Logical Operator29/1
  Logical Operator26/1 -> S-R Flip-Flop4/2
  Logical Operator25/1 -> Logical Operator29/2
  Logical Operator36/1 -> Logical Operator35/2
  Logical Operator24/1 -> Logical Operator28/1
  Logical Operator31/1 -> Logical Operator26/2
  Logical Operator16/1 -> Logical Operator20/1
  Logical Operator35/1 -> S-R Flip-Flop5/1
  Logical Operator21/1 -> Logical Operator20/2
  Logical Operator19/1 -> S-R Flip-Flop3/1
  Logical Operator18/1 -> S-R Flip-Flop3/2
  Logical Operator29/1 -> Logical Operator28/2
  Logical Operator32/1 -> Logical Operator36/1
  Logical Operator37/1 -> Logical Operator36/2
  S-R Flip-Flop3/1 -> Button 1/1
  Logical Operator40/1 -> Logical Operator44/1
  Logical Operator45/1 -> Logical Operator44/2
  Logical Operator20/1 -> Logical Operator19/2
  Logical Operator43/1 -> S-R Flip-Flop6/1
  Logical Operator44/1 -> Logical Operator43/2
  Logical Operator27/1 -> S-R Flip-Flop4/1
  Logical Operator28/1 -> Logical Operator27/2
  S-R Flip-Flop5/1 -> Button 2/1
  S-R Flip-Flop6/1 -> Button 3/1
  S-R Flip-Flop4/1 -> Button 4/1

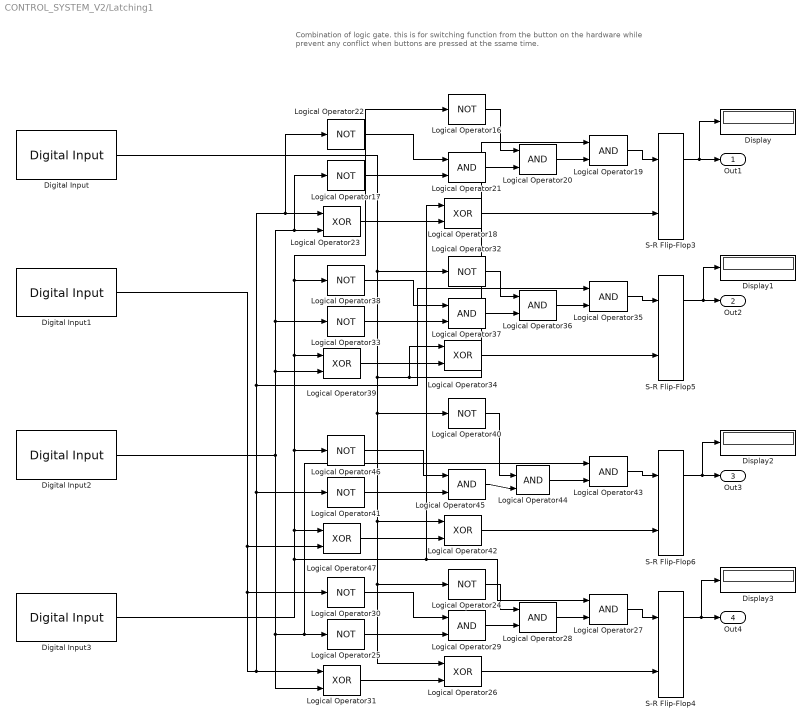
== system CONTROL_SYSTEM_V2/Latching1 ==
  note: Combination of logic gate. this is for switching function from the button on the hardware while prevent any conflict when buttons are pressed at the ssame time.
  Digital Input : arduinolib/Digital Input  pinNumber=36  mode=Default  Direction=input  SampleTime=-1  blockPlatform=arduino
  Digital Input1 : arduinolib/Digital Input  pinNumber=39  mode=Default  Direction=input  SampleTime=-1  blockPlatform=arduino
  Digital Input2 : arduinolib/Digital Input  pinNumber=34  mode=Default  Direction=input  SampleTime=-1  blockPlatform=arduino
  Digital Input3 : arduinolib/Digital Input  pinNumber=35  mode=Default  Direction=input  SampleTime=-1  blockPlatform=arduino
  Display{,1..3} (4 alike) : Display
  Logical Operator{16..17,22,24..25,30,32..33,38,40..41,46} (12 alike) : Logic  Operator=NOT  IconShape=distinctive  AllPortsSameDT=off  OutDataTypeStr=boolean
  Logical Operator{18,23,26,31,34,39,42,47} (8 alike) : Logic  Operator=XOR  IconShape=distinctive  AllPortsSameDT=off  OutDataTypeStr=boolean
  Logical Operator{19..21,27..29,35..37,43..45} (12 alike) : Logic  IconShape=distinctive  AllPortsSameDT=off  OutDataTypeStr=boolean
  S-R Flip-Flop{3..6} (4 alike) : simulink_extras/Flip Flops/S-R Flip-Flop  initial_condition=0
  Out1 : Outport
  Out2 : Outport  Port=2
  Out3 : Outport  Port=3
  Out4 : Outport  Port=4
  wires:
  Digital Input2/1 -> Logical Operator25/1, Logical Operator43/1, Logical Operator31/2, Logical Operator17/1, Logical Operator23/2, Logical Operator33/1, Logical Operator39/2
  Digital Input3/1 -> Logical Operator16/1, Logical Operator38/1, Logical Operator39/1, Logical Operator46/1, Logical Operator47/1, Logical Operator18/1, Logical Operator27/1
  Digital Input1/1 -> Logical Operator47/2, Logical Operator30/1, Logical Operator41/1, Logical Operator22/1, Logical Operator23/1, Logical Operator35/1, Logical Operator31/1
  Logical Operator22/1 -> Logical Operator21/1
  Logical Operator17/1 -> Logical Operator21/2
  Logical Operator34/1 -> S-R Flip-Flop5/2
  Logical Operator33/1 -> Logical Operator37/2
  Logical Operator23/1 -> Logical Operator18/2
  Logical Operator39/1 -> Logical Operator34/2
  Logical Operator38/1 -> Logical Operator37/1
  Digital Input/1 -> Logical Operator40/1, Logical Operator24/1, Logical Operator26/1, Logical Operator42/1, Logical Operator19/1, Logical Operator34/1, Logical Operator32/1
  Logical Operator47/1 -> Logical Operator42/2
  Logical Operator46/1 -> Logical Operator45/1
  Logical Operator42/1 -> S-R Flip-Flop6/2
  Logical Operator41/1 -> Logical Operator45/2
  Logical Operator30/1 -> Logical Operator29/1
  Logical Operator26/1 -> S-R Flip-Flop4/2
  Logical Operator25/1 -> Logical Operator29/2
  Logical Operator36/1 -> Logical Operator35/2
  Logical Operator24/1 -> Logical Operator28/1
  Logical Operator31/1 -> Logical Operator26/2
  Logical Operator16/1 -> Logical Operator20/1
  Logical Operator35/1 -> S-R Flip-Flop5/1
  Logical Operator21/1 -> Logical Operator20/2
  Logical Operator19/1 -> S-R Flip-Flop3/1
  Logical Operator18/1 -> S-R Flip-Flop3/2
  Logical Operator29/1 -> Logical Operator28/2
  Logical Operator32/1 -> Logical Operator36/1
  Logical Operator37/1 -> Logical Operator36/2
  S-R Flip-Flop3/1 -> Display/1, Out1/1
  Logical Operator40/1 -> Logical Operator44/1
  Logical Operator45/1 -> Logical Operator44/2
  Logical Operator20/1 -> Logical Operator19/2
  Logical Operator43/1 -> S-R Flip-Flop6/1
  Logical Operator44/1 -> Logical Operator43/2
  Logical Operator27/1 -> S-R Flip-Flop4/1
  Logical Operator28/1 -> Logical Operator27/2
  S-R Flip-Flop5/1 -> Display1/1, Out2/1
  S-R Flip-Flop6/1 -> Display2/1, Out3/1
  S-R Flip-Flop4/1 -> Display3/1, Out4/1

== system CONTROL_SYSTEM_V2/No Control ==
  In1 : Inport
  Action Port : ActionPort  ActionPortLabel=if(u1 == 1)
  Out1 : Outport
  wires:
  In1/1 -> Out1/1

== system CONTROL_SYSTEM_V2/Operation Selector ==
  note: As the output of button is binary, therefore there are either 0 or 1. the simple equation for this is (Button_1 * 1) + (Button_2 * 2) + (Button_3 * 3) = Desired Mode
  note: Switch condition:
      | If the first button is pressed (output = 1), the system will run "No Control" mode
      | If the second button is pressed (output = 2), the system will run "PID Control" Mode
      | If the third button is pressed (output = 3), the system will run "Advanced Control" Mode
  No Control : Inport
  PID Output : Inport  Port=2
  Advanced Control : Inport  Port=3
  Switch 1 : Inport  Port=4
  Switch 2 : Inport  Port=5
  Switch 3 : Inport  Port=6
  Add : Sum  Inputs=+++
  Multiply : Gain
  Multiply1 : Gain  Gain=2
  Multiply2 : Gain  Gain=3
  Multiport Switch : MultiPortSwitch  DiagnosticForDefault=None  SaturateOnIntegerOverflow=off  InputSameDT=off
  Control Output : Outport
  wires:
  No Control/1 -> Multiport Switch/2
  Multiply/1 -> Add/1
  Multiply2/1 -> Add/3
  Add/1 -> Multiport Switch/1
  Switch 1/1 -> Multiply/1
  Multiply1/1 -> Add/2
  Switch 2/1 -> Multiply1/1
  Switch 3/1 -> Multiply2/1
  Advanced Control/1 -> Multiport Switch/4
  PID Output/1 -> Multiport Switch/3
  Multiport Switch/1 -> Control Output/1

== system CONTROL_SYSTEM_V2/PID Control ==
  note: PID control, with the saturation block to control the integral wind-up or any over shooting
      | the value of 0.01 is to give a room for slight over shooting value
  Error : Inport
  FP_maxVal : Inport  Port=2
  FP_minVal : Inport  Port=3
  Action Port : ActionPort  ActionPortLabel=elseif(u2 == 1)
  Constant : Constant  Value=0.01
  PID Controller2 : slpidlib/PID Controller  Controller=PID  Form=Parallel  TimeDomain=Continuous-time  UseExternalTs=off  SampleTime=-1  IntegratorMethod=Forward Euler  FilterMethod=Forward Euler  ControllerParametersSource=internal  P=Kp  I=Ki  UseKiTs=off  D=Kd  UseExternalDerivativeSource=off  N=Kn  UseFilter=on  TunerSelectOption=Transfer Function Based (PID Tuner App)  InitialConditionSource=internal  InitialConditionForIntegrator=0  InitialConditionForFilter=0  DifferentiatorICPrevScaledInput=0  ExternalReset=none  TrackingMode=off  Kt=1  LimitOutput=off  SatLimitsSource=internal  UpperSaturationLimit=inf  LowerSaturationLimit=-inf  LinearizeAsGain=on  AntiWindupMode=none  Kb=1  LimitIntegrator=off  UpperIntegratorSaturationLimit=inf  LowerIntegratorSaturationLimit=-inf  POutMin=[]  POutMax=[]  IOutMin=[]  IOutMax=[]  DOutMin=[]  DOutMax=[]  NOutMin=[]  NOutMax=[]  SumOutMin=[]  SumOutMax=[]  SaturationOutMin=[]  SaturationOutMax=[]  PParamMin=[]  PParamMax=[]  IParamMin=[]  IParamMax=[]  DParamMin=[]  DParamMax=[]  NParamMin=[]  NParamMax=[]  KbParamMin=[]  KbParamMax=[]  KtParamMin=[]  KtParamMax=[]  KbOutMin=[]  KbOutMax=[]  KtOutMin=[]  KtOutMax=[]  IntegratorOutMin=[]  IntegratorOutMax=[]  FilterOutMin=[]  FilterOutMax=[]  SumI1OutMin=[]  SumI1OutMax=[]  SumI2OutMin=[]  SumI2OutMax=[]  SumI3OutMin=[]  SumI3OutMax=[]  SumI4OutMin=[]  SumI4OutMax=[]  SumDOutMin=[]  SumDOutMax=[]  DifferentiatorOutMin=[]  DifferentiatorOutMax=[]  FilterDiffOutCoefMin=[]  FilterDiffOutCoefMax=[]  ReciprocalOutMin=[]  ReciprocalOutMax=[]  SumDenOutMin=[]  SumDenOutMax=[]  SumNumOutMin=[]  SumNumOutMax=[]  DivideOutMin=[]  DivideOutMax=[]  UdiffTsProdOutMin=[]  UdiffTsProdOutMax=[]  NTsProdOutMin=[]  NTsProdOutMax=[]  UintegralTsProdOutMin=[]  UintegralTsProdOutMax=[]  UngainTsProdOutMin=[]  UngainTsProdOutMax=[]  ClampingZeroOutDataTypeStr=Inherit: Inherit via back propagation  ClampingZeroOutMin=[]  ClampingZeroOutMax=[]  FilterDenConstantOutDataTypeStr=Inherit: Inherit via back propagation  FilterDenConstantOutMin=[]  FilterDenConstantOutMax=[]  PCopyOutDataTypeStr=Inherit: Inherit via back propagation  PCopyOutMin=[]  PCopyOutMax=[]  NCopyOutDataTypeStr=Inherit: Inherit via back propagation  NCopyOutMin=[]  NCopyOutMax=[]  IntegratorContinuousStateAttributes=''  IntegratorStateMustResolveToSignalObject=off  IntegratorRTWStateStorageClass=Auto  FilterContinuousStateAttributes=''  FilterStateMustResolveToSignalObject=off  FilterRTWStateStorageClass=Auto  ParallelPVariant=InternalParameters  IdealPVariant=Disabled  IVariant=InternalParameters  DVariant=InternalParameters  IntegratorVariant=Continuous  SatVariant=Disabled  AWVariant=Passthrough  PCopyVariant=Disabled  TRVariant=Disabled  FdbkBlocksVariant=Forward  IdealPFdbkVariant=Disabled  SatFdbkVariant=Disabled  DerivativeFilterVariant=ContFilter  NVariant=InternalParameters  NCopyVariant=Disabled  FilterICVariant=InternalICsFilter  IntegratorICVariant=InternalICs  ExternalResetVariant=Disabled  TRSumVariant=Passthrough  SumFdbkVariant=Disabled  SumVariant=Sum_PID  TsampFilterVariant=InternalTs  TsampNgainVariant=Passthrough  TsampIntegralVariant=Disabled_SignalSpec  ExternalSaturationOutDataTypeStr=Inherit: Same as second input  DerivativeSourceVariant=ErrorSignal
  Saturation Dynamic : simulink/Discontinuities/Saturation Dynamic  OutMin=[]  OutMax=[]  OutDataTypeStr=Inherit: Same as second input  OutDataType=fixdt(1, 16)  OutScaling=2^-10  DoSatur=off
  Sum1 : Sum  Inputs=++|
  PID Output : Outport
  wires:
  Saturation Dynamic/1 -> PID Output/1
  FP_minVal/1 -> Saturation Dynamic/3
  Error/1 -> PID Controller2/1
  PID Controller2/1 -> Saturation Dynamic/2
  Sum1/1 -> Saturation Dynamic/1
  Constant/1 -> Sum1/1
  FP_maxVal/1 -> Sum1/2

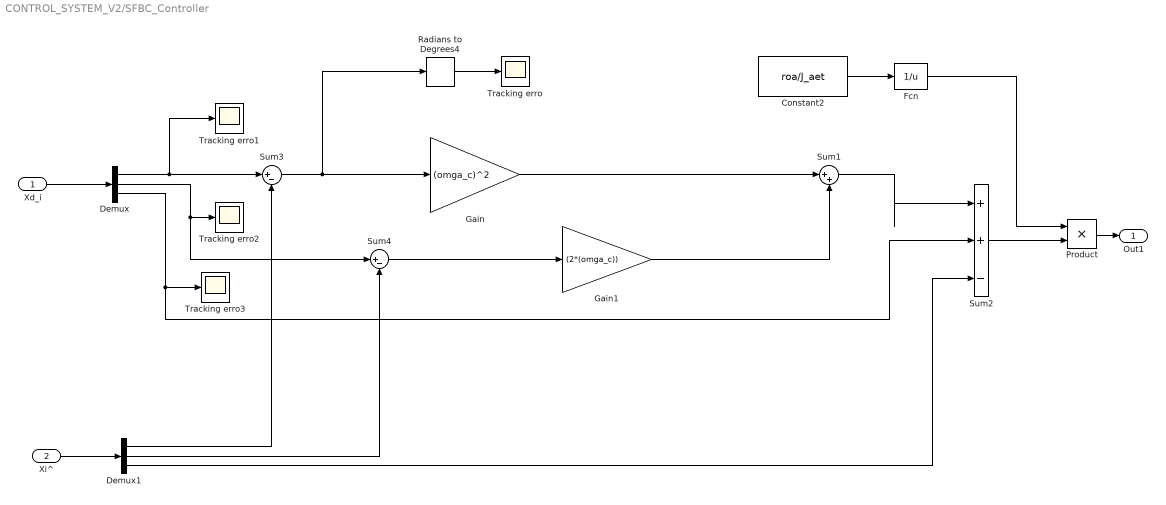
== system CONTROL_SYSTEM_V2/SFBC_Controller ==
  Xd_i : Inport
  Xi^ : Inport  Port=2
  Constant2 : Constant  Value=roa/J_aet
  Demux : Demux  Outputs=3
  Demux1 : Demux  Outputs=3
  Fcn : Fcn  Expr=1/u
  Gain : Gain  Gain=(omga_c)^2
  Gain1 : Gain  Gain=(2*(omga_c))
  Product : Product  RndMeth=Zero
  Radians to Degrees4 : simulink_extras/Transformations/Radians to Degrees
  Sum1 : Sum  Inputs=|++
  Sum2 : Sum  Inputs=|++-
  Sum3 : Sum  Inputs=|+-
  Sum4 : Sum  Inputs=|+-
  Tracking erro{,1..3} (4 alike) : Scope
  Out1 : Outport
  wires:
  Gain/1 -> Sum1/1
  Gain1/1 -> Sum1/2
  Sum1/1 -> Sum2/1
  Constant2/1 -> Fcn/1
  Fcn/1 -> Product/1
  Sum2/1 -> Product/2
  Demux1/3 -> Sum2/3
  Product/1 -> Out1/1
  Demux/3 -> Tracking erro3/1, Sum2/2
  Sum4/1 -> Gain1/1
  Xd_i/1 -> Demux/1
  Demux/1 -> Tracking erro1/1, Sum3/1
  Xi^/1 -> Demux1/1
  Demux1/1 -> Sum3/2
  Demux/2 -> Tracking erro2/1, Sum4/1
  Demux1/2 -> Sum4/2
  Sum3/1 -> Radians to Degrees4/1, Gain/1
  Radians to Degrees4/1 -> Tracking erro/1

== system CONTROL_SYSTEM_V2/Subsystem ==
  Throttle Body Feedback : Inport
  In1 : Inport  Port=2
  Abs : Abs  SaturateOnIntegerOverflow=off
  Divide : Product  Inputs=*/
  Gain : Gain  Gain=100
  Percentage Error : Outport
  wires:
  Divide/1 -> Abs/1
  Gain/1 -> Percentage Error/1  "Percentage Error"
  Abs/1 -> Gain/1
  In1/1 -> Divide/1
  Throttle Body Feedback/1 -> Divide/2

== system CONTROL_SYSTEM_V2/Subsystem1 ==
  In1 : Inport
  Pedal_Val : Inport  Port=2
  Constant : Constant  Value=0
  Constant1 : Constant
  Constant2 : Constant  Value=0.02
  Detect Increase1 : simulink/Logic and Bit Operations/Detect Increase  vinit=0.0  OutDataTypeStr=boolean
  Display13 : Display
      settings: Decimation=2
  MATLAB Function : MATLAB Function  TreatAsAtomicUnit=on
  Relational Operator : RelationalOperator  OutDataTypeStr=boolean  RndMeth=Simplest  InputSameDT=off
  Switch : Switch  Criteria=u2 ~= 0  Threshold=1  SaturateOnIntegerOverflow=off  InputSameDT=off
  Desire_Val : Outport
  wires:
  MATLAB Function/1(Desire_Val) -> Desire_Val/1
  In1/1 -> Relational Operator/2
  Switch/1 -> Display13/1, [try]
  Detect Increase1/1 -> Switch/2
  Constant/1 -> Switch/1
  Constant2/1 -> Relational Operator/1
  Constant1/1 -> Switch/3
  Relational Operator/1 -> Detect Increase1/1
  Pedal_Val/1 -> MATLAB Function/1(Pedal_Val)
